simulink model "tank_pos_pos_2022a"  (R2022a)
settings: Solver=VariableStepAuto  StartTime=0.0  StopTime=10.0  RelTol=1e-3
values from neighbouring files (symbols this model uses):
  A = 1    [tank_force_pos_params.m]    (also in tank_pos_pos_params.m)
  alpha = 0.1    [tank_force_pos_params.m]    (also in tank_pos_pos_params.m = 0.2)
  Be = 100    [tank_force_pos_params.m]    (also in tank_pos_pos_params.m)
  beta = 0.1    [tank_force_pos_params.m]    (also in tank_pos_pos_params.m = 0.01)
  Bh = 1.5    [tank_force_pos_params.m]    (also in tank_pos_pos_params.m)
  Bm = 10    [tank_force_pos_params.m]    (also in tank_pos_pos_params.m)
  Bs = 10    [tank_force_pos_params.m]    (also in tank_pos_pos_params.m)
  delay = 10    [tank_force_pos_params.m]    (also in tank_pos_pos_params.m = 100)
  Dh = 20*0.8    (= 16)    [tank_force_pos_params.m]    (also in tank_pos_pos_params.m)
  Fc = 0.5    [tank_force_pos_params.m]    (also in tank_pos_pos_params.m)
  Flp = 5    [tank_force_pos_params.m]    (also in tank_pos_pos_params.m)
  H_D = 100    [tank_force_pos_params.m]    (also in tank_pos_pos_params.m)
  initial_tank_energy_master = 100 * 10    (= 1000)    [tank_force_pos_params.m]    (also in tank_pos_pos_params.m)
  initial_tank_energy_slave = 100 * 10    (= 1000)    [tank_force_pos_params.m]    (also in tank_pos_pos_params.m)
  Jh = 1    [tank_force_pos_params.m]    (also in tank_pos_pos_params.m)
  Ke = 200    [tank_force_pos_params.m]    (also in tank_pos_pos_params.m)
  Km = 50    [tank_force_pos_params.m]    (also in tank_pos_pos_params.m)
  Ks = 50    [tank_force_pos_params.m]    (also in tank_pos_pos_params.m)
  Mm = 0.5    [tank_force_pos_params.m]    (also in tank_pos_pos_params.m)
  Ms = 2    [tank_force_pos_params.m]    (also in tank_pos_pos_params.m)
  Ph = 10*1    (= 10)    [tank_force_pos_params.m]    (also in tank_pos_pos_params.m)
  Ts = 0.001    [tank_force_pos_params.m]    (also in tank_pos_pos_params.m)
  xe = 0.5    [tank_force_pos_params.m]    (also in tank_pos_pos_params.m = 5)
settings Model: Creator=Manu  LastModifiedBy=Manu
settings ModelReferenceCC: EnableRefExpFcnMdlSchedulingChecks=off
settings RTWCC: Description=Generic Real-Time Target

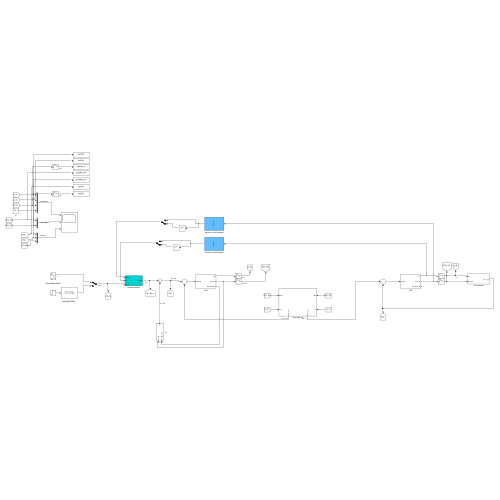
[thumbnail: Simulink's stored preview of the top-level diagram]
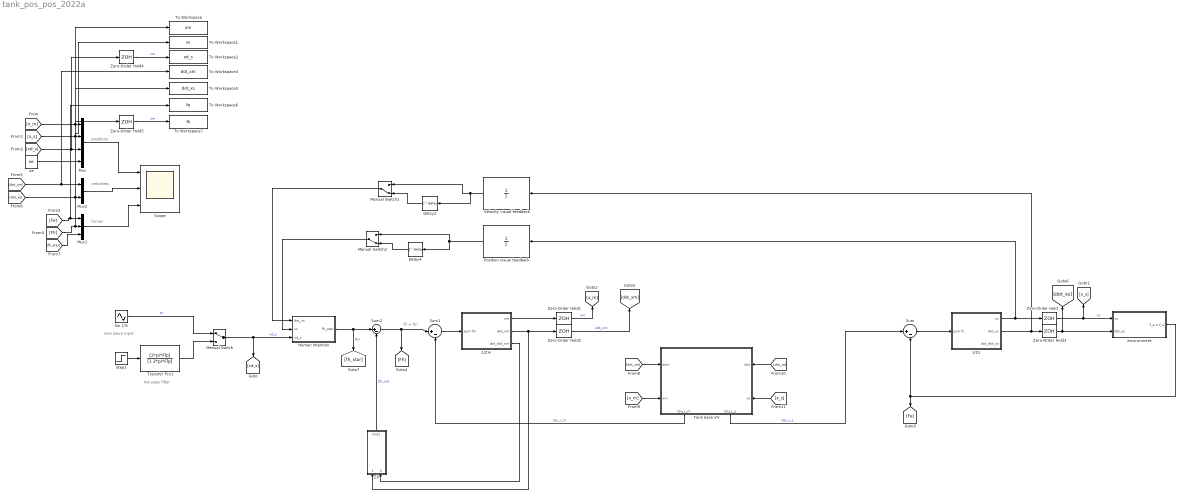
== system tank_pos_pos_2022a ==
  note: fh = fm
  note: sine wave input
  note: low pass filter
  note: forces
  note: positions
  note: velocities
  1/Zm : Subsystem
  1/Zs : Subsystem
  Delay2 : Delay  DelayLength=delay  SampleTime=Ts
  Delay4 : Delay  DelayLength=delay  SampleTime=Ts
  Human Intention : Subsystem
  Manual Switch : ManualSwitch
  Manual Switch1 : ManualSwitch  CurrentSetting=0
  Manual Switch2 : ManualSwitch  CurrentSetting=0
  Mux : Mux
  Mux1 : Mux  Inputs=3
  Mux2 : Mux  Inputs=2
  Position visual feedback : TransferFcn  Denominator=[1]
  Scope : Scope  NumInputPorts=3
  Sin 17t : Sin  Amplitude=A  Frequency=2*pi*Fc  SampleTime=0
  Step1 : Step  Time=0.5  After=A  SampleTime=0
  Sum : Sum  Inputs=|+-
  Sum1 : Sum  Inputs=|+-
  Sum2 : Sum  Inputs=|+-
  Tank base VV : Subsystem
      settings: PortSchema="{\"entries\":[{\"content\":{\"sides\":[{\"content\":{\"connectorIds\":[\"In1\",\"In2\"]},\"type\":\"ConnectorPlacement.EquallySpacedRectSide\",\"uuid\":\"3a964002-fb37-4a92-b745-35f358b8e187\"},{\"content\":{\"connectorIds\":[\"In3\",\"In4\"],\"side\":\"RIGHT\"},\"type\":\"ConnectorPlacement.EquallySpacedRectSide\",\"uuid\":\"6a0ade08-0aa0-46a3-9e09-c310668c505c\"},{\"content\":{\"connectorIds\":[],\"side\":\"TOP\"},\"type\":\"ConnectorPlacement.EquallySpacedRectSide\",\"uuid\":\"1dfd7bbc-8185-4b5f-95de-42c58388ee02\"},{\"content\":{\"connectorIds\":[\"Out1\",\"Out2\"],\"side\":\"BOTTOM\"},\"type\":\"ConnectorPlacement.EquallySpacedRectSide\",\"uuid\":\"8c57ed43-4006-4572-ac50-c9adf88e8601\"},{\"content\":{\"connectorIds\":[],\"side\":\"HIDDEN\"},\"type\":\"ConnectorPlacement.EquallySpacedRectSide\",\"uuid\":\"15175a08-ca5b-4167-ba1d-f2e8cd3d814b\"}]},\"type\":\"ConnectorPlacement.EquallySpacedConnector\",\"uuid\":\"2bd1e993-3bc7-4875-9b20-3fb59092d5ec\"}],\"packageUris\":[\"http://schema.mathworks.com/mf0/Connector/R2020b\"],\"version\":\"1.0\"}"
  To Workspace : ToWorkspace  VariableName=xm  SaveFormat=Timeseries  SampleTime=-1
  To Workspace1 : ToWorkspace  VariableName=xs  SaveFormat=Timeseries  SampleTime=-1
  To Workspace2 : ToWorkspace  VariableName=xd_s  SaveFormat=Timeseries  SampleTime=-1
  To Workspace4 : ToWorkspace  VariableName=dot_xm  SaveFormat=Timeseries  SampleTime=-1
  To Workspace5 : ToWorkspace  VariableName=dot_xs  SaveFormat=Timeseries  SampleTime=-1
  To Workspace6 : ToWorkspace  VariableName=fe  SaveFormat=Timeseries  SampleTime=-1
  To Workspace7 : ToWorkspace  VariableName=fh  SaveFormat=Timeseries  SampleTime=-1
  Transfer Fcn1 : TransferFcn  Numerator=[2*pi*Flp]  Denominator=[1 2*pi*Flp]
  Velocity visual feedback : TransferFcn  Denominator=[1]
  Zero-Order Hold{,1..5} (6 alike) : ZeroOrderHold  SampleTime=Ts
  Zh : Subsystem
  environment : Subsystem
  xe : Constant  Value=xe
  wires:
  1/Zm/1(xm) -> Zero-Order Hold1/1
  Manual Switch/1 -> Human Intention/3(xd_s), [xd_s]  "xd_s"
  Zh/1(Out1) -> Sum2/2  "Zh_out"
  Sin 17t/1 -> Manual Switch/1  "F*"
  1/Zm/3(dot_dot_xm) -> Zh/2(dot_dot_xm)
  Human Intention/1(fh_star) -> Sum2/1, [fh_star]  "fh*"
  Transfer Fcn1/1 -> Manual Switch/2
  Step1/1 -> Transfer Fcn1/1
  Sum2/1 -> [Fh], Sum1/1
  Sum1/1 -> 1/Zm/1(sum fm)
  Sum/1 -> 1/Zs/1(sum fs)
  1/Zs/2(dot_xs) -> Velocity visual feedback/1, Zero-Order Hold3/1
  1/Zs/1(xs) -> Zero-Order Hold/1, Position visual feedback/1
  environment/1(f_e = f_s) -> [Fe], Sum/2
  Velocity visual feedback/1 -> Delay2/1, Manual Switch1/1
  Manual Switch1/1 -> Human Intention/1(dot_xs)
  Delay4/1 -> Manual Switch2/2
  Position visual feedback/1 -> Delay4/1, Manual Switch2/1
  Manual Switch2/1 -> Human Intention/2(xs)
  1/Zm/2(dot_xm) -> Zero-Order Hold2/1, Zh/1(dot_xm)
  Delay2/1 -> Manual Switch1/2
  Zero-Order Hold1/1 -> [x_m]  "xm"
  Zero-Order Hold2/1 -> [dot_xm]  "dot_xm"
  Tank base VV/1(tau_r_m) -> Sum1/2  "tau_r_m"
  [x_m] -> Tank base VV/2(xm)
  [dot_xm] -> Tank base VV/1(dxm)
  [dot_xs] -> Tank base VV/3(dxs)
  [x_s] -> Tank base VV/4(xs)
  Tank base VV/2(tau_r_s) -> Sum/1  "tau_r_s"
  Zero-Order Hold/1 -> [x_s], environment/1(xs)  "xs"
  Zero-Order Hold3/1 -> [dot_xs], environment/2(dot_xs)
  [xd_s] -> Zero-Order Hold4/1, Mux/3
  [fh_star] -> Mux1/3
  [x_m] -> To Workspace/1, Mux/1
  xe/1 -> Mux/4
  Mux/1 -> Scope/1
  Mux1/1 -> Scope/3
  [Fe] -> Mux1/1, To Workspace6/1
  [dot_xm] -> Mux2/1, To Workspace4/1
  Mux2/1 -> Scope/2
  [x_s] -> To Workspace1/1, Mux/2
  [Fh] -> Zero-Order Hold5/1, Mux1/2
  [dot_xs] -> To Workspace5/1, Mux2/2
  Zero-Order Hold4/1 -> To Workspace2/1  "xm"
  Zero-Order Hold5/1 -> To Workspace7/1  "xm"

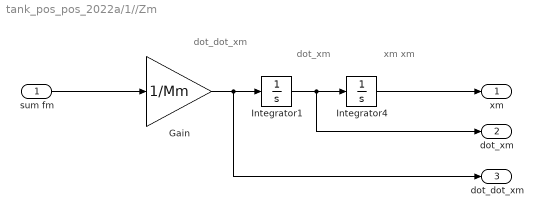
== system tank_pos_pos_2022a/1//Zm ==
  note: dot_dot_xm
  note: dot_xm
  note: xm
      | xm
  sum fm : Inport
  Gain : Gain  Gain=1/Mm
  Integrator1 : Integrator
  Integrator4 : Integrator
  xm : Outport
  dot_xm : Outport  Port=2
  dot_dot_xm : Outport  Port=3
  wires:
  sum fm/1 -> Gain/1
  Gain/1 -> dot_dot_xm/1, Integrator1/1
  Integrator4/1 -> xm/1
  Integrator1/1 -> dot_xm/1, Integrator4/1

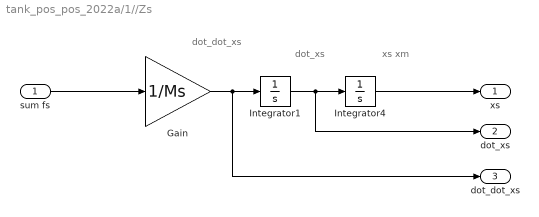
== system tank_pos_pos_2022a/1//Zs ==
  note: dot_dot_xs
  note: dot_xs
  note: xs
      | xm
  sum fs : Inport
  Gain : Gain  Gain=1/Ms
  Integrator1 : Integrator
  Integrator4 : Integrator
  xs : Outport
  dot_xs : Outport  Port=2
  dot_dot_xs : Outport  Port=3
  wires:
  sum fs/1 -> Gain/1
  Gain/1 -> dot_dot_xs/1, Integrator1/1
  Integrator4/1 -> xs/1
  Integrator1/1 -> dot_xs/1, Integrator4/1

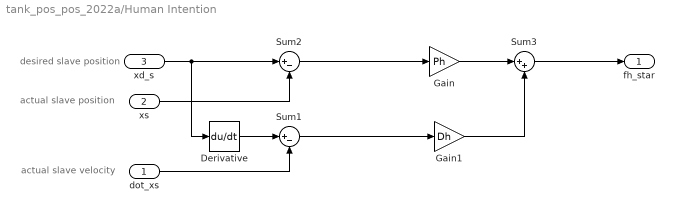
== system tank_pos_pos_2022a/Human Intention ==
  note: actual slave velocity
  note: actual slave position
  note: desired slave position
  dot_xs : Inport
  xs : Inport  Port=2
  xd_s : Inport  Port=3
  Derivative : Derivative
  Gain : Gain  Gain=Ph
  Gain1 : Gain  Gain=Dh
  Sum1 : Sum  Inputs=|+-
  Sum2 : Sum  Inputs=|+-
  Sum3 : Sum  Inputs=|++
  fh_star : Outport
  wires:
  xs/1 -> Sum2/2
  dot_xs/1 -> Sum1/2
  Sum2/1 -> Gain/1
  Sum1/1 -> Gain1/1
  Gain1/1 -> Sum3/2
  Gain/1 -> Sum3/1
  Sum3/1 -> fh_star/1
  xd_s/1 -> Derivative/1, Sum2/1
  Derivative/1 -> Sum1/1

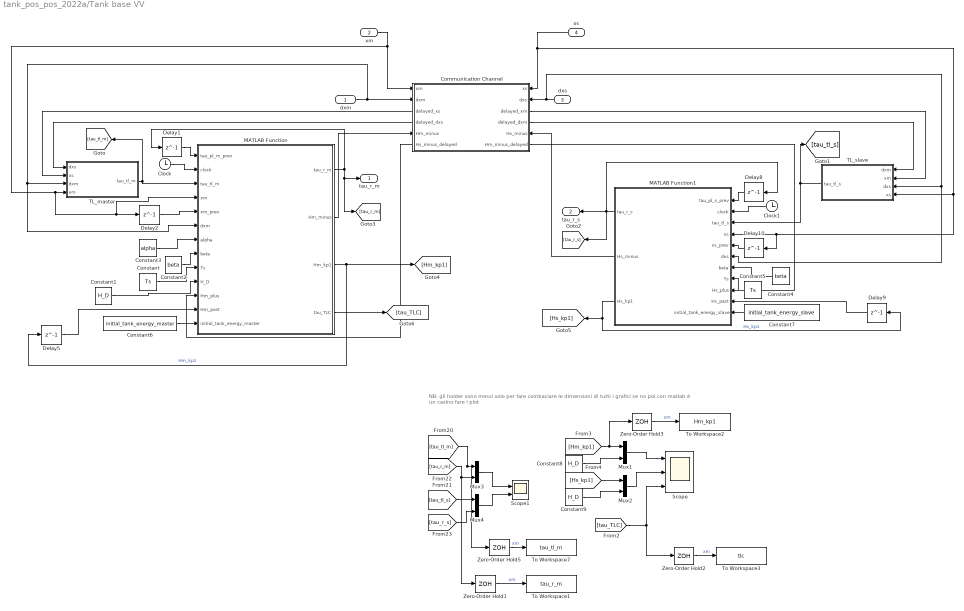
== system tank_pos_pos_2022a/Tank base VV ==
  note: NB: gli holder sono messi solo per fare combaciare le dimensioni di tutti i grafici se no poi con matlab è un casino fare i plot
  dxm : Inport
  xm : Inport  Port=2
  dxs : Inport  Port=3
  xs : Inport  Port=4
  Clock : Clock
  Clock1 : Clock
  Communication Channel : Subsystem
      settings: PortSchema="{\"entries\":[{\"content\":{\"sides\":[{\"content\":{\"connectorIds\":[\"In1\",\"In2\",\"Out4\",\"Out5\",\"In3\",\"Out6\"]},\"type\":\"ConnectorPlacement.EquallySpacedRectSide\",\"uuid\":\"707b854d-ad7a-498f-bed1-9a4f8657ce88\"},{\"content\":{\"connectorIds\":[\"In4\",\"In5\",\"Out1\",\"Out2\",\"In6\",\"Out3\"],\"side\":\"RIGHT\"},\"type\":\"ConnectorPlacement.EquallySpacedRectSide\",\"uuid\":\"12f3e034-857d-4081-a3d0-204c7e32b1d7\"},{\"content\":{\"connectorIds\":[],\"side\":\"TOP\"},\"type\":\"ConnectorPlacement.EquallySpacedRectSide\",\"uuid\":\"fb6b09f7-6084-4258-a6c2-180f375b33c2\"},{\"content\":{\"connectorIds\":[],\"side\":\"HIDDEN\"},\"type\":\"ConnectorPlacement.EquallySpacedRectSide\",\"uuid\":\"424096ec-dcd8-463d-bba6-855fd00452bd\"}]},\"type\":\"ConnectorPlacement.EquallySpacedConnector\",\"uuid\":\"13b09cb8-9f61-41a9-b654-31f5f7de73c5\"}],\"packageUris\":[\"http://schema.mathworks.com/mf0/Connector/R2020b\"],\"version\":\"1.0\"}"
  Constant : Constant  Value=Ts
  Constant1 : Constant  Value=H_D
  Constant2 : Constant  Value=beta
  Constant3 : Constant  Value=alpha
  Constant4 : Constant  Value=beta
  Constant5 : Constant  Value=Ts
  Constant6 : Constant  Value=initial_tank_energy_master
  Constant7 : Constant  Value=initial_tank_energy_slave
  Constant8 : Constant  Value=H_D
  Constant9 : Constant  Value=H_D
  Delay{1..2,5,8..10} (6 alike) : Delay  DelayLength=1
  MATLAB Function : MATLAB Function  TreatAsAtomicUnit=on
  MATLAB Function1 : MATLAB Function  TreatAsAtomicUnit=on
  Mux{1..4} (4 alike) : Mux  Inputs=2
  Scope : Scope  NumInputPorts=3
  Scope1 : Scope  NumInputPorts=2
  TL_master : Subsystem
  TL_slave : Subsystem
  To Workspace1 : ToWorkspace  VariableName=tau_r_m  SaveFormat=Timeseries  SampleTime=-1
  To Workspace2 : ToWorkspace  VariableName=Hm_kp1  SaveFormat=Timeseries  SampleTime=-1
  To Workspace3 : ToWorkspace  VariableName=tlc  SaveFormat=Timeseries  SampleTime=-1
  To Workspace7 : ToWorkspace  VariableName=tau_tl_m  SaveFormat=Timeseries  SampleTime=-1
  Zero-Order Hold{1..3,5} (4 alike) : ZeroOrderHold  SampleTime=Ts
  tau_r_m : Outport
  tau_r_s : Outport  Port=2
  wires:
  TL_master/1(tau_tl_m) -> [tau_tl_m], MATLAB Function/3(tau_tl_m)
  Clock/1 -> MATLAB Function/2(clock)
  MATLAB Function/1(tau_r_m) -> [tau_r_m], tau_r_m/1, Delay1/1
  Delay1/1 -> MATLAB Function/1(tau_pl_m_prev)
  Delay2/1 -> MATLAB Function/5(xm_prev)
  Delay5/1 -> MATLAB Function/12(Hm_past)
  Constant/1 -> MATLAB Function/9(Ts)
  Constant1/1 -> MATLAB Function/10(H_D)
  MATLAB Function/3(Hm_kp1) -> Delay5/1, [Hm_kp1]  "Hm_kp1"
  Constant2/1 -> MATLAB Function/8(beta)
  Constant3/1 -> MATLAB Function/7(alpha)
  Communication Channel/3(Hs_minus_delayed) -> MATLAB Function/11(Hm_plus)
  MATLAB Function1/1(tau_r_s) -> Delay8/1, [tau_r_s], tau_r_s/1
  Delay8/1 -> MATLAB Function1/1(tau_pl_s_prev)
  Clock1/1 -> MATLAB Function1/2(clock)
  Constant4/1 -> MATLAB Function1/7(beta)
  Constant5/1 -> MATLAB Function1/8(Ts)
  Delay9/1 -> MATLAB Function1/10(Hs_past)
  MATLAB Function1/3(Hs_kp1) -> Delay9/1, [Hs_kp1]  "Hs_kp1"
  Delay10/1 -> MATLAB Function1/5(xs_prev)
  xs/1 -> Communication Channel/1(xs), Delay10/1, MATLAB Function1/4(xs), TL_slave/4(xs)
  xm/1 -> Communication Channel/4(xm), MATLAB Function/4(xm), Delay2/1, TL_master/4(xm)
  dxm/1 -> MATLAB Function/6(dxm), TL_master/3(dxm), Communication Channel/5(dxm)
  dxs/1 -> Communication Channel/2(dxs), MATLAB Function1/6(dxs), TL_slave/3(dxs)
  MATLAB Function/2(Hm_minus) -> Communication Channel/6(Hm_minus)
  MATLAB Function1/2(Hs_minus) -> Communication Channel/3(Hs_minus)
  Communication Channel/6(Hm_minus_delayed) -> MATLAB Function1/9(Hs_plus)
  Communication Channel/4(delayed_xm) -> TL_slave/2(xm)
  Communication Channel/5(delayed_dxm) -> TL_slave/1(dxm)
  Communication Channel/1(delayed_xs) -> TL_master/2(xs)
  Communication Channel/2(delayed_dxs) -> TL_master/1(dxs)
  TL_slave/1(tau_tl_s) -> [tau_tl_s], MATLAB Function1/3(tau_tl_s)
  Constant6/1 -> MATLAB Function/13(initial_tank_energy_master)
  Constant7/1 -> MATLAB Function1/11(initial_tank_energy_slave)
  Mux4/1 -> Scope1/2
  [tau_tl_m] -> Zero-Order Hold5/1, Mux3/1
  [tau_tl_s] -> Mux4/1
  [tau_r_s] -> Mux4/2
  Mux3/1 -> Scope1/1
  [tau_r_m] -> Mux3/2, Zero-Order Hold1/1
  MATLAB Function/4(tau_TLC) -> [tau_TLC]
  [tau_TLC] -> Zero-Order Hold2/1, Scope/3
  [Hm_kp1] -> Mux1/1, Zero-Order Hold3/1
  [Hs_kp1] -> Mux2/1
  Constant8/1 -> Mux1/2
  Constant9/1 -> Mux2/2
  Mux1/1 -> Scope/1
  Mux2/1 -> Scope/2
  Zero-Order Hold5/1 -> To Workspace7/1  "xm"
  Zero-Order Hold1/1 -> To Workspace1/1  "xm"
  Zero-Order Hold2/1 -> To Workspace3/1  "xm"
  Zero-Order Hold3/1 -> To Workspace2/1  "xm"

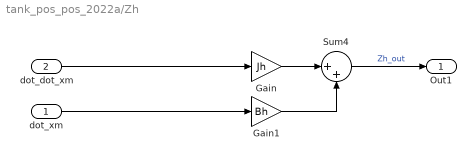
== system tank_pos_pos_2022a/Zh ==
  dot_xm : Inport
  dot_dot_xm : Inport  Port=2
  Gain : Gain  Gain=Jh
  Gain1 : Gain  Gain=Bh
  Sum4 : Sum  Inputs=|++
  Out1 : Outport
  wires:
  dot_dot_xm/1 -> Gain/1
  Gain1/1 -> Sum4/2
  Gain/1 -> Sum4/1
  Sum4/1 -> Out1/1  "Zh_out"
  dot_xm/1 -> Gain1/1

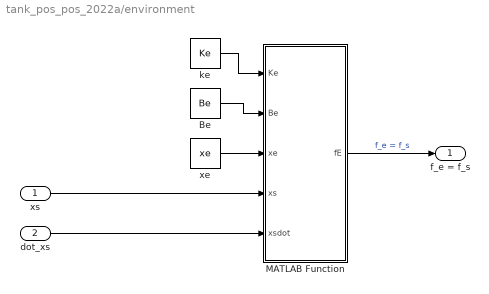
== system tank_pos_pos_2022a/environment ==
  xs : Inport
  dot_xs : Inport  Port=2
  Be : Constant  Value=Be
  MATLAB Function : MATLAB Function  TreatAsAtomicUnit=on
  ke : Constant  Value=Ke
  xe : Constant  Value=xe
  f_e = f_s : Outport
  wires:
  MATLAB Function/1(fE) -> f_e = f_s/1  "f_e = f_s"
  xs/1 -> MATLAB Function/4(xs)
  xe/1 -> MATLAB Function/3(xe)
  dot_xs/1 -> MATLAB Function/5(xsdot)
  ke/1 -> MATLAB Function/1(Ke)
  Be/1 -> MATLAB Function/2(Be)

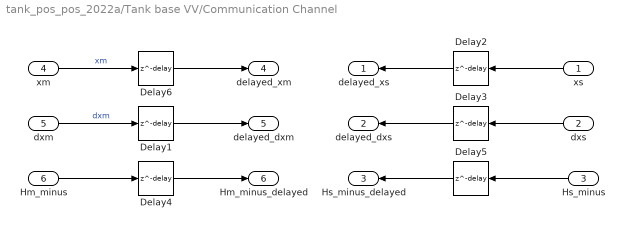
== system tank_pos_pos_2022a/Tank base VV/Communication Channel ==
  xs : Inport
  dxs : Inport  Port=2
  Hs_minus : Inport  Port=3
  xm : Inport  Port=4
  dxm : Inport  Port=5
  Hm_minus : Inport  Port=6
  Delay{1..6} (6 alike) : Delay  DelayLength=delay  SampleTime=Ts
  delayed_xs : Outport
  delayed_dxs : Outport  Port=2
  Hs_minus_delayed : Outport  Port=3
  delayed_xm : Outport  Port=4
  delayed_dxm : Outport  Port=5
  Hm_minus_delayed : Outport  Port=6
  wires:
  xm/1 -> Delay6/1  "xm"
  dxm/1 -> Delay1/1  "dxm"
  Delay6/1 -> delayed_xm/1
  Delay1/1 -> delayed_dxm/1
  Delay3/1 -> delayed_dxs/1
  xs/1 -> Delay2/1
  dxs/1 -> Delay3/1
  Delay2/1 -> delayed_xs/1
  Hm_minus/1 -> Delay4/1
  Delay4/1 -> Hm_minus_delayed/1
  Delay5/1 -> Hs_minus_delayed/1
  Hs_minus/1 -> Delay5/1

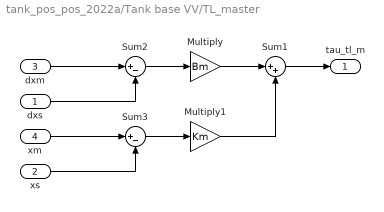
== system tank_pos_pos_2022a/Tank base VV/TL_master ==
  dxs : Inport
  xs : Inport  Port=2
  dxm : Inport  Port=3
  xm : Inport  Port=4
  Multiply : Gain  Gain=Bm
  Multiply1 : Gain  Gain=Km
  Sum1 : Sum  Inputs=|++
  Sum2 : Sum  Inputs=|+-
  Sum3 : Sum  Inputs=|+-
  tau_tl_m : Outport
  wires:
  Sum2/1 -> Multiply/1
  Multiply1/1 -> Sum1/2
  Multiply/1 -> Sum1/1
  Sum1/1 -> tau_tl_m/1
  Sum3/1 -> Multiply1/1
  xm/1 -> Sum3/1
  dxm/1 -> Sum2/1
  xs/1 -> Sum3/2
  dxs/1 -> Sum2/2

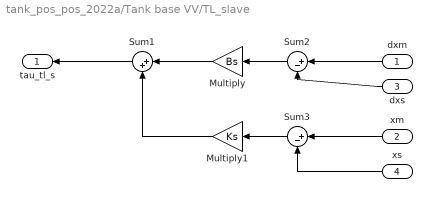
== system tank_pos_pos_2022a/Tank base VV/TL_slave ==
  dxm : Inport
  xm : Inport  Port=2
  dxs : Inport  Port=3
  xs : Inport  Port=4
  Multiply : Gain  Gain=Bs
  Multiply1 : Gain  Gain=Ks
  Sum1 : Sum  Inputs=|++
  Sum2 : Sum  Inputs=|+-
  Sum3 : Sum  Inputs=|+-
  tau_tl_s : Outport
  wires:
  Sum2/1 -> Multiply/1
  Multiply1/1 -> Sum1/2
  Multiply/1 -> Sum1/1
  Sum1/1 -> tau_tl_s/1
  Sum3/1 -> Multiply1/1
  xs/1 -> Sum3/2
  dxs/1 -> Sum2/2
  xm/1 -> Sum3/1
  dxm/1 -> Sum2/1

== matlab function tank_pos_pos_2022a/Tank base VV/MATLAB Function ==
  data: tau_pl_m_prev input; clock input; tau_r_m output; Hm_minus output; tau_tl_m input; xm input; xm_prev input; dxm input; alpha input; beta input; Ts input; H_D input; Hm_plus input; Hm_past input; Hm_kp1 output; initial_tank_energy_master input; tau_TLC output
function [tau_r_m, Hm_minus, Hm_kp1, tau_TLC] = passivity_layer_master(tau_pl_m_prev, clock, tau_tl_m, xm, xm_prev, dxm, alpha, beta, Ts, H_D, Hm_plus, Hm_past, initial_tank_energy_master)
    if clock == 0
        Hm_past = initial_tank_energy_master;
        tau_pl_m_prev = 0;
        xm_prev = 0; 
    end
    
    delta_xm = xm - xm_prev;
    delta_H_used = tau_pl_m_prev*(delta_xm);
    Hm_k = Hm_past + Hm_plus - delta_H_used;

    
    % Computation of H_kp1
    
    % Send energy
    if (Hm_k > 0)
        Hm_minus =  beta*Hm_k;
        Hm_kp1 = Hm_k - Hm_minus;  
    else
        Hm_minus = 0;
        Hm_kp1 = 0;
    end
    
    % TLC check
    if(Hm_kp1 < H_D)
       % H_D - Hm_kp1 = di quanto siamo sotto soglia
       d = alpha*(H_D - Hm_kp1);
       tau_TLC = -d*dxm;
    else
       tau_TLC = 0;
    end
    
    % Compute tau limits
    if Hm_kp1 <= 0 
        tau_max_m_1 = 0;
    else
        tau_max_m_1 = tau_tl_m;
    end
    
%     if abs(dxm) < 0.001
%         tau_max_m_2 = 1e3;
%     else
        tau_max_m_2 =  Hm_kp1/(dxm*Ts);
%     end
    
    tau_pl_m = sign(tau_tl_m)*min([abs(tau_tl_m), abs(tau_max_m_1), abs(tau_max_m_2)]);
    
    tau_r_m = tau_pl_m + tau_TLC;

end

== matlab function tank_pos_pos_2022a/environment/MATLAB Function ==
  data: Ke input; fE output; Be input; xe input; xs input; xsdot input
function fE = environment(Ke, Be, xe, xs, xsdot)
    if xs > xe
        fE = Ke * (xs - xe) + Be * xsdot; % Plot both contributions Ke and Be
    else
        fE = 0;
    end
end

== matlab function tank_pos_pos_2022a/Tank base VV/MATLAB Function1 ==
  data: tau_r_s output; Hs_minus output; tau_pl_s_prev input; Hs_kp1 output; clock input; tau_tl_s input; xs input; xs_prev input; dxs input; beta input; Ts input; Hs_plus input; Hs_past input; initial_tank_energy_slave input
function [tau_r_s, Hs_minus, Hs_kp1 ] = passivity_layer_slave(tau_pl_s_prev, clock, tau_tl_s, xs, xs_prev, dxs, beta, Ts, Hs_plus, Hs_past, initial_tank_energy_slave)
    if clock == 0
        Hs_past = initial_tank_energy_slave;
        tau_pl_s_prev = 0;
        xs_prev = 0;
    end
    
    delta_xs = xs - xs_prev;
    delta_H_used = tau_pl_s_prev*(delta_xs);
    Hs_k = Hs_past + Hs_plus - delta_H_used;
 
    % Send energy
    if (Hs_k > 0)
        Hs_minus =  beta*Hs_k;
        Hs_kp1 = Hs_k - Hs_minus;  
    else
        Hs_kp1 = 0;
        Hs_minus = 0;
    end
    
    % Compute tau limits
    if Hs_kp1 <= 0 
        tau_max_s_1 = 0;
    else
        tau_max_s_1 = tau_tl_s;
    end
    
%     if abs(dxs) < 0.001
%         tau_max_s_2 = 1e3;
%     else
        tau_max_s_2 =  Hs_kp1/(dxs*Ts);
%     end
    
    tau_pl_s = sign(tau_tl_s)*min([abs(tau_tl_s), abs(tau_max_s_1), abs(tau_max_s_2)]);
    
    tau_r_s = tau_pl_s;
    
   
end
